simulink model "stage1_profiled_loop_model"  (R2026a)
settings: Solver=ode45  StopTime=0.5
undefined symbols (not defined in the file): B, CPR, J, Ke, Kt, L, R, TL, Ts_disc, V_dc
settings Model: Creator=knavn  LastModifiedBy=knavn

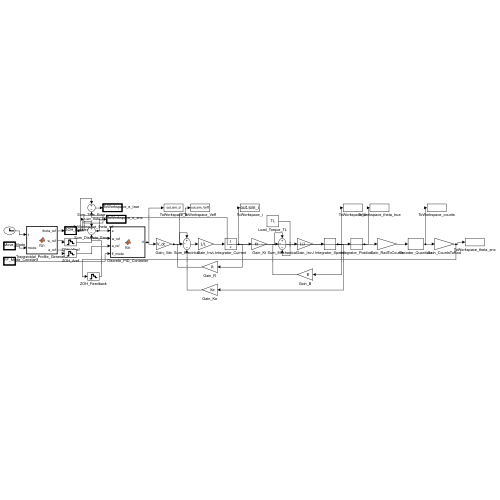
[thumbnail: Simulink's stored preview of the top-level diagram]
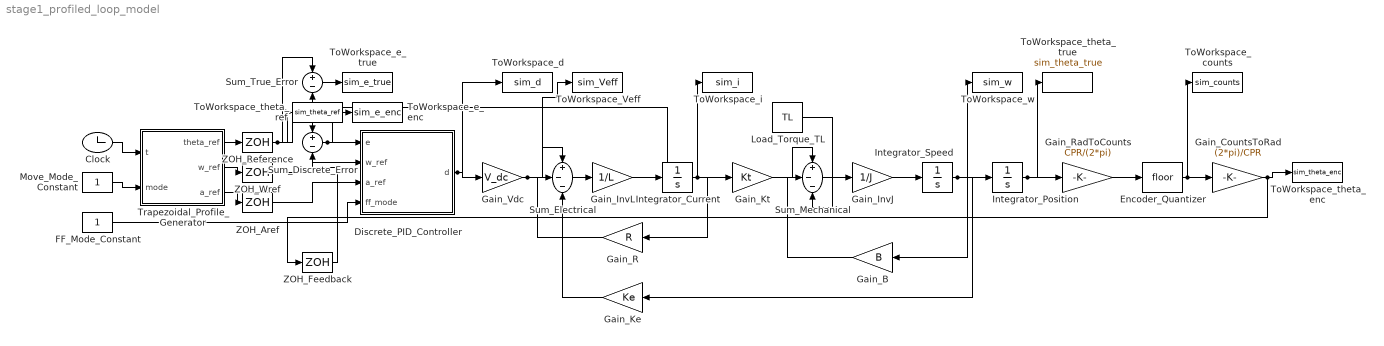
== system stage1_profiled_loop_model ==
  Clock : Clock
  Discrete_PID_Controller : MATLAB Function  TreatAsAtomicUnit=on
  Encoder_Quantizer : Rounding
  FF_Mode_Constant : Constant
  Gain_B : Gain  Gain=B
  Gain_CountsToRad : Gain  Gain=(2*pi)/CPR
  Gain_InvJ : Gain  Gain=1/J
  Gain_InvL : Gain  Gain=1/L
  Gain_Ke : Gain  Gain=Ke
  Gain_Kt : Gain  Gain=Kt
  Gain_R : Gain  Gain=R
  Gain_RadToCounts : Gain  Gain=CPR/(2*pi)
  Gain_Vdc : Gain  Gain=V_dc
  Integrator_Current : Integrator
  Integrator_Position : Integrator
  Integrator_Speed : Integrator
  Load_Torque_TL : Constant  Value=TL
  Move_Mode_Constant : Constant
  Sum_Discrete_Error : Sum  Inputs=+-
  Sum_Electrical : Sum  Inputs=+--
  Sum_Mechanical : Sum  Inputs=+--
  Sum_True_Error : Sum  Inputs=+-
  ToWorkspace_Veff : ToWorkspace  VariableName=sim_Veff  SaveFormat=Timeseries  SampleTime=-1
  ToWorkspace_counts : ToWorkspace  VariableName=sim_counts  SaveFormat=Timeseries  SampleTime=-1
  ToWorkspace_d : ToWorkspace  VariableName=sim_d  SaveFormat=Timeseries  SampleTime=-1
  ToWorkspace_e_enc : ToWorkspace  VariableName=sim_e_enc  SaveFormat=Timeseries  SampleTime=-1
  ToWorkspace_e_true : ToWorkspace  VariableName=sim_e_true  SaveFormat=Timeseries  SampleTime=-1
  ToWorkspace_i : ToWorkspace  VariableName=sim_i  SaveFormat=Timeseries  SampleTime=-1
  ToWorkspace_theta_enc : ToWorkspace  VariableName=sim_theta_enc  SaveFormat=Timeseries  SampleTime=-1
  ToWorkspace_theta_ref : ToWorkspace  VariableName=sim_theta_ref  SaveFormat=Timeseries  SampleTime=-1
  ToWorkspace_theta_true : ToWorkspace  VariableName=sim_theta_true  SaveFormat=Timeseries  SampleTime=-1
  ToWorkspace_w : ToWorkspace  VariableName=sim_w  SaveFormat=Timeseries  SampleTime=-1
  Trapezoidal_Profile_Generator : MATLAB Function  TreatAsAtomicUnit=on
  ZOH_Aref : ZeroOrderHold  SampleTime=Ts_disc
  ZOH_Feedback : ZeroOrderHold  SampleTime=Ts_disc
  ZOH_Reference : ZeroOrderHold  SampleTime=Ts_disc
  ZOH_Wref : ZeroOrderHold  SampleTime=Ts_disc
  wires:
  Clock/1 -> Trapezoidal_Profile_Generator/1(t)
  Move_Mode_Constant/1 -> Trapezoidal_Profile_Generator/2(mode)
  Trapezoidal_Profile_Generator/1(theta_ref) -> ZOH_Reference/1
  Trapezoidal_Profile_Generator/2(w_ref) -> ZOH_Wref/1
  Trapezoidal_Profile_Generator/3(a_ref) -> ZOH_Aref/1
  ZOH_Reference/1 -> Sum_Discrete_Error/1, Sum_True_Error/1, ToWorkspace_theta_ref/1
  Sum_True_Error/1 -> ToWorkspace_e_true/1
  Sum_Discrete_Error/1 -> Discrete_PID_Controller/1(e), ToWorkspace_e_enc/1
  ZOH_Wref/1 -> Discrete_PID_Controller/2(w_ref)
  ZOH_Aref/1 -> Discrete_PID_Controller/3(a_ref)
  FF_Mode_Constant/1 -> Discrete_PID_Controller/4(ff_mode)
  Discrete_PID_Controller/1(d) -> Gain_Vdc/1, ToWorkspace_d/1
  Gain_Vdc/1 -> Sum_Electrical/1, ToWorkspace_Veff/1
  Sum_Electrical/1 -> Gain_InvL/1
  Gain_InvL/1 -> Integrator_Current/1
  Integrator_Current/1 -> Gain_R/1, Gain_Kt/1, ToWorkspace_i/1
  Gain_R/1 -> Sum_Electrical/2
  Gain_Kt/1 -> Sum_Mechanical/1
  Load_Torque_TL/1 -> Sum_Mechanical/3
  Sum_Mechanical/1 -> Gain_InvJ/1
  Gain_InvJ/1 -> Integrator_Speed/1
  Integrator_Speed/1 -> Gain_B/1, Gain_Ke/1, Integrator_Position/1, ToWorkspace_w/1
  Gain_B/1 -> Sum_Mechanical/2
  Gain_Ke/1 -> Sum_Electrical/3
  Integrator_Position/1 -> Sum_True_Error/2, ToWorkspace_theta_true/1, Gain_RadToCounts/1
  Gain_RadToCounts/1 -> Encoder_Quantizer/1
  Encoder_Quantizer/1 -> ToWorkspace_counts/1, Gain_CountsToRad/1
  Gain_CountsToRad/1 -> ToWorkspace_theta_enc/1, ZOH_Feedback/1
  ZOH_Feedback/1 -> Sum_Discrete_Error/2

== matlab function stage1_profiled_loop_model/Discrete_PID_Controller ==
  data: e input; d output; w_ref input; a_ref input; ff_mode input
function d = Discrete_PID_Controller(e, w_ref, a_ref, ff_mode)
% Corrected Discrete PID Controller (Ts = 1 ms) - Validated Optimization
% Kp=0.50, Ki=8.00, Kd=0.0000, N=20 with Conditional Anti-Windup Clamping
if ff_mode == 0 % Phase 1 Unassisted Baseline Failed Configuration
    Kp = 2.50;
    Ki = 0.50;
    Kd = 0.080;
    N  = 100;
    Kff_v = 0.0;
    Kff_a = 0.0;
else % Phase 2 Corrected & Validated Optimized Feedforward Configuration
    Kp = 0.50;
    Ki = 8.00;
    Kd = 0.0000;
    N  = 20;
    Kff_v = 0.004175;             % (Ke + R*B/Kt) / V_dc
    Kff_a = 0.00000834;           % (J*R/Kt + L*B/Kt) / V_dc
end
Ts = 0.001;

persistent u_i u_d e_prev
if isempty(u_i)
    u_i = 0.0;
    u_d = 0.0;
    e_prev = 0.0;
end

% 1. Discrete Proportional Term
u_p = Kp * e;

% 2. Discrete Derivative Term (Backward Euler with Filter N)
u_d = (Kd * N * (e - e_prev) + u_d) / (1.0 + N * Ts);

% 3. Tentative Discrete Integrator Update
v_i = u_i + Ki * Ts * e;

% 4. Explicit Configurable Feedforward Term
if ff_mode == 1
    u_ff = Kff_v * w_ref + Kff_a * a_ref;
else
    u_ff = 0.0;
end

% 5. Total Tentative Control Output u_calc
u_calc = u_p + v_i + u_d + u_ff;

% 6. Actuator Duty Cycle Saturation [0.0, 1.0]
if u_calc > 1.0
    d = 1.0;
elseif u_calc < 0.0
    d = 0.0;
else
    d = u_calc;
end

% 7. Conditional Integration Anti-Windup Clamping
is_sat_high = (u_calc > 1.0) && (e > 0);
is_sat_low  = (u_calc < 0.0) && (e < 0);
if is_sat_high || is_sat_low
    u_i = u_i;
else
    u_i = v_i;
end

e_prev = e;
end

== matlab function stage1_profiled_loop_model/Trapezoidal_Profile_Generator ==
  data: t input; theta_ref output; mode input; w_ref output; a_ref output
function [theta_ref, w_ref, a_ref] = Trapezoidal_Profile_Generator(t, mode)
% Kinematic Trapezoidal Profile Generator for Stage 1 Step 5
a_max = 50.0; % rad/s^2
w_max = 8.0;  % rad/s
step_rad = 90.0 * pi / 180; % 1.5707963 rad
t_a = w_max / a_max; % 0.160 s
theta_a = 0.5 * a_max * t_a^2; % 0.640 rad
t_c = (step_rad - 2 * theta_a) / w_max; % 0.0363495 s
t_f = 2 * t_a + t_c; % 0.3563495 s

if mode == 1 % Single 90 deg Indexing Move
    t_start = 0.050;
    [theta_ref, w_ref, a_ref] = calc_single_move(t, t_start, step_rad, a_max, w_max, t_a, theta_a, t_c, t_f);
else % 3x Sequential 90 deg Indexing Moves (0 -> 90 -> 180 -> 270 deg)
    t_start1 = 0.050;
    t_start2 = 0.500;
    t_start3 = 0.950;
    [th1, w1, a1] = calc_single_move(t, t_start1, step_rad, a_max, w_max, t_a, theta_a, t_c, t_f);
    [th2, w2, a2] = calc_single_move(t, t_start2, step_rad, a_max, w_max, t_a, theta_a, t_c, t_f);
    [th3, w3, a3] = calc_single_move(t, t_start3, step_rad, a_max, w_max, t_a, theta_a, t_c, t_f);
    theta_ref = th1 + th2 + th3;
    w_ref = w1 + w2 + w3;
    a_ref = a1 + a2 + a3;
end
end

function [th, w, a] = calc_single_move(t, t_start, step_rad, a_max, w_max, t_a, theta_a, t_c, t_f)
if t < t_start
    th = 0.0; w = 0.0; a = 0.0;
elseif t < t_start + t_a
    dt = t - t_start;
    th = 0.5 * a_max * dt^2;
    w = a_max * dt;
    a = a_max;
elseif t < t_start + t_a + t_c
    dt = t - t_start - t_a;
    th = theta_a + w_max * dt;
    w = w_max;
    a = 0.0;
elseif t < t_start + t_f
    dt = t_start + t_f - t;
    th = step_rad - 0.5 * a_max * dt^2;
    w = a_max * dt;
    a = -a_max;
else
    th = step_rad;
    w = 0.0;
    a = 0.0;
end
end
